simulink subsystem "duty_cycle_allocation_mT_PWM_2"  (R2020b)
settings: Solver=VariableStepAuto  StartTime=0.0  StopTime=10.0  RelTol=1e-3
undefined symbols (not defined in the file): T_PWM_1, T_PWM_2
settings Model: Creator=leop9  LastModifiedBy=Previ

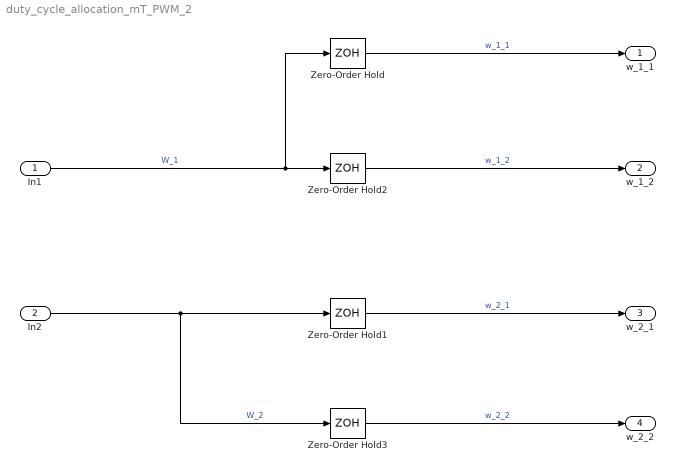
== system duty_cycle_allocation_mT_PWM_2 ==
  In1 : Inport
  In2 : Inport  Port=2
  Zero-Order Hold : ZeroOrderHold  SampleTime=T_PWM_1
  Zero-Order Hold1 : ZeroOrderHold  SampleTime=T_PWM_1
  Zero-Order Hold2 : ZeroOrderHold  SampleTime=T_PWM_2
  Zero-Order Hold3 : ZeroOrderHold  SampleTime=T_PWM_2
  w_1_1 : Outport
  w_1_2 : Outport  Port=2
  w_2_1 : Outport  Port=3
  w_2_2 : Outport  Port=4
  wires:
  In1/1 -> Zero-Order Hold/1, Zero-Order Hold2/1  "W_1"
  In2/1 -> Zero-Order Hold3/1, Zero-Order Hold1/1  "W_2"
  Zero-Order Hold2/1 -> w_1_2/1  "w_1_2"
  Zero-Order Hold/1 -> w_1_1/1  "w_1_1"
  Zero-Order Hold3/1 -> w_2_2/1  "w_2_2"
  Zero-Order Hold1/1 -> w_2_1/1  "w_2_1"
